simulink model "Simulator_hquad_LQR_trajectory"  (Simulink 7.6)
settings: Solver=ode3  StartTime=0.0  StopTime=40  FixedStep=Ts  RelTol=1e-3
values from neighbouring files (symbols this model uses):
  g = 9.8065    [kostas_malakies.mat]    (also in kostas_malakies2.mat; load_PMModel.m = 9.81; main_last.m; matlab.mat)
  mass = 0.66    [kostas_malakies.mat]    (also in kostas_malakies2.mat; load_PMModel.m = 0.687; main_last.m)
  Ts = 0.02    [kostas_malakies.mat]    (also in kostas_malakies2.mat; main.m; main_last.m; matlab.mat = 0.08)
  Ts_slow = 0.02    [kostas_malakies.mat]    (also in kostas_malakies2.mat; main.m; main_last.m)
  yaw0 = 0    [kostas_malakies.mat]    (also in kostas_malakies2.mat; main.m; main_last.m; matlab.mat = -0.0873)
libraries: simulink x14, Hqaud_model_LIB_SI x5, Hquad_control_LIB_LQR x5, sdolib x4
settings Model: Creator=andi  LastModifiedBy=burrimi
settings DebuggingCC: InheritedTsInSrcMsg=none  StrictBusMsg=Warning
settings SFSimCC: SimParseCustomCode=off

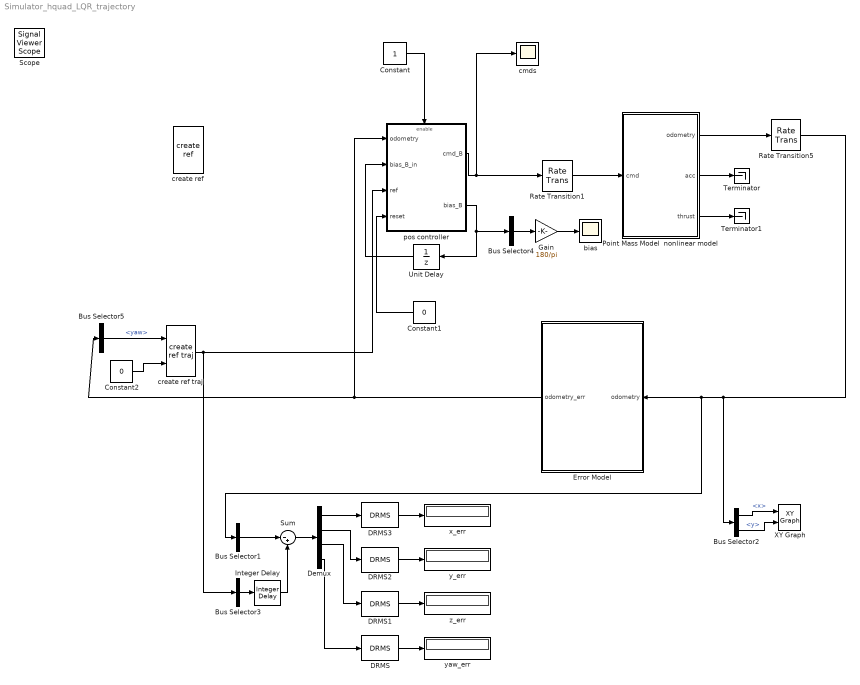
== system Simulator_hquad_LQR_trajectory ==
  Bus Selector1 : BusSelector  OutputSignals=pos.x,pos.y,pos.z,rpy.yaw  OutputAsBus=on
  Bus Selector2 : BusSelector  OutputSignals=pos.x,pos.y
  Bus Selector3 : BusSelector  OutputSignals=x_ref,y_ref,z_ref,yaw_ref  OutputAsBus=on
  Bus Selector4 : BusSelector  OutputSignals=pitch_bias,roll_bias,thrust_bias  OutputAsBus=on
  Bus Selector5 : BusSelector  OutputSignals=rpy.yaw
  Constant : Constant
  Constant1 : Constant  Value=0
  Constant2 : Constant  Value=0
  DRMS{,1..3} (4 alike) : sdolib/RMS Blocks/DRMS  SystemSampleTime=-1  Ts=Ts
  Demux : Demux
  Error Model : Subsystem
  Gain : Gain  Gain=180/pi
  Integer Delay : simulink/Discrete/Integer Delay  NumDelays=3  vinit=0.0  samptime=-1
  Point Mass Model  nonlinear model : Subsystem  AncestorBlock="Hqaud_model_LIB_SI/Point Mass Model  nonlinear model"
  Rate Transition1 : RateTransition
  Rate Transition5 : RateTransition  OutPortSampleTime=Ts
  Sum : Sum  Inputs=|-+
  Terminator : Terminator
  Terminator1 : Terminator
  Unit Delay : UnitDelay  SampleTime=-1
  XY Graph : simulink/Sinks/XY Graph  SystemSampleTime=-1  xmin=-2  xmax=2  ymin=-2  ymax=2  st=-1
  bias : Scope
      settings: TimeRange=39.996  YMin=-0.07  YMax=0.05  SaveName=ScopeData14
  cmds : Scope
      settings: TimeRange=40  YMin=-0.5  YMax=0.5
  create ref : Hquad_control_LIB_LQR/create ref  SystemSampleTime=-1
  create ref traj : Hquad_control_LIB_LQR/create ref traj  SystemSampleTime=-1
  pos controller : Subsystem  AncestorBlock=Hquad_control_LIB_LQR/pos controller
  x_err : Display
  y_err : Display
  yaw_err : Display
  z_err : Display
  Scope : SignalViewerScope  IOType=viewer  LegendLocations="321.25       180.625         123.5       128.125"  RefreshTime=0.035000
      settings: ShowLegends=on
  wires:
  Point Mass Model  nonlinear model/3("thrust   ") -> Terminator1/1
  pos controller/1(cmd_B) -> cmds/1, Rate Transition1/1
  Constant/1 -> pos controller/Enable
  Point Mass Model  nonlinear model/2(acc) -> Terminator/1
  Constant1/1 -> pos controller/4(reset)
  Point Mass Model  nonlinear model/1(odometry) -> Rate Transition5/1
  Error Model/1(odometry_err) -> Bus Selector5/1, pos controller/1(odometry)
  Rate Transition5/1 -> Bus Selector2/1, Error Model/1(odometry), Bus Selector1/1
  Bus Selector1/1 -> Sum/1
  Sum/1 -> Demux/1
  Demux/1 -> DRMS3/1
  Demux/2 -> DRMS2/1
  Demux/3 -> DRMS1/1
  Demux/4 -> DRMS/1
  DRMS/1 -> yaw_err/1
  DRMS1/1 -> z_err/1
  DRMS2/1 -> y_err/1
  DRMS3/1 -> x_err/1
  Rate Transition1/1 -> Point Mass Model  nonlinear model/1(cmd)
  Bus Selector3/1 -> Integer Delay/1
  Bus Selector5/1 -> create ref traj/1  "<yaw>"
  pos controller/2(bias_B) -> Unit Delay/1, Bus Selector4/1
  Bus Selector4/1 -> Gain/1
  Gain/1 -> bias/1
  Unit Delay/1 -> pos controller/2(bias_B_in)
  create ref traj/1 -> Bus Selector3/1, pos controller/3(ref)
  Bus Selector2/1 -> XY Graph/1  "<x>"
  Bus Selector2/2 -> XY Graph/2  "<y>"
  Integer Delay/1 -> Sum/2
  Constant2/1 -> create ref traj/2

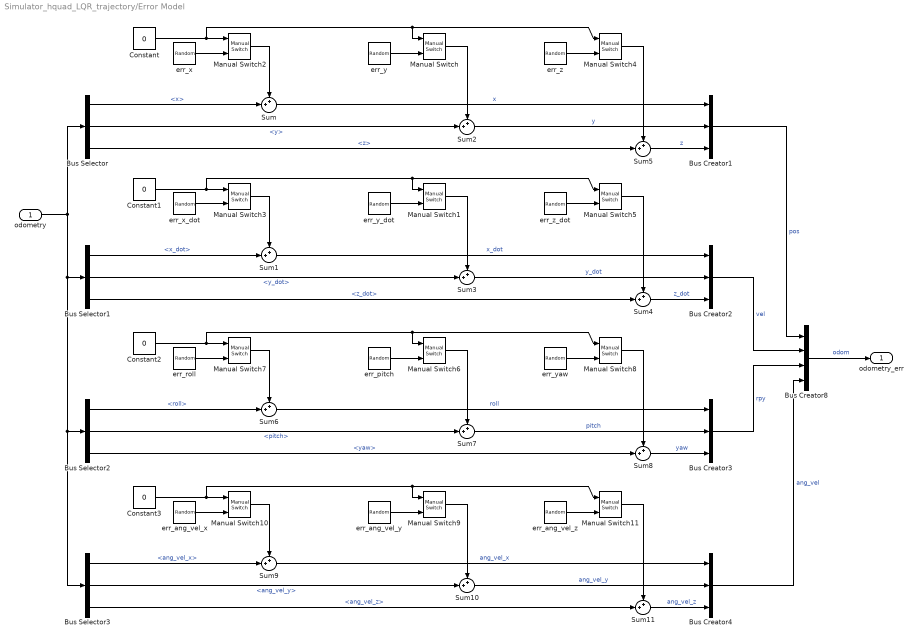
== system Simulator_hquad_LQR_trajectory/Error Model ==
  odometry : Inport
  Bus Creator{1..4} (4 alike) : BusCreator  Inputs=3
  Bus Creator8 : BusCreator
  Bus Selector : BusSelector  OutputSignals=pos.x,pos.y,pos.z
  Bus Selector1 : BusSelector  OutputSignals=vel.x_dot,vel.y_dot,vel.z_dot
  Bus Selector2 : BusSelector  OutputSignals=rpy.roll,rpy.pitch,rpy.yaw
  Bus Selector3 : BusSelector  OutputSignals=ang_vel.ang_vel_x,ang_vel.ang_vel_y,ang_vel.ang_vel_z
  Constant{,1..3} (4 alike) : Constant  Value=0
  Manual Switch{,1..11} (12 alike) : simulink/Signal Routing/Manual Switch  SystemSampleTime=-1  sw=1  action=0  varsize=off
  Sum{,1..11} (12 alike) : Sum  Inputs=++|  SampleTime=Ts_slow
  err_ang_vel_x : RandomNumber  Variance=0.0001  SampleTime=Ts_slow
  err_ang_vel_y : RandomNumber  Variance=0.0001  SampleTime=Ts_slow
  err_ang_vel_z : RandomNumber  Variance=0.0001  SampleTime=Ts_slow
  err_pitch : RandomNumber  Variance=0.0001  SampleTime=Ts_slow
  err_roll : RandomNumber  Variance=0.0001  SampleTime=Ts_slow
  err_x : RandomNumber  Variance=0.000707  SampleTime=Ts_slow
  err_x_dot : RandomNumber  Variance=0.0001  SampleTime=Ts_slow
  err_y : RandomNumber  Variance=0.000707  SampleTime=Ts_slow
  err_y_dot : RandomNumber  Variance=0.0001  SampleTime=Ts_slow
  err_yaw : RandomNumber  Variance=0.0001  SampleTime=Ts_slow
  err_z : RandomNumber  Variance=0.000707  SampleTime=Ts_slow
  err_z_dot : RandomNumber  Variance=0.0001  SampleTime=Ts_slow
  odometry_err : Outport
  wires:
  err_z/1 -> Manual Switch4/2
  Manual Switch4/1 -> Sum5/1
  err_y/1 -> Manual Switch/2
  Manual Switch/1 -> Sum2/1
  err_x/1 -> Manual Switch2/2
  Manual Switch2/1 -> Sum/1
  Sum/1 -> Bus Creator1/1  "x"
  Bus Creator1/1 -> Bus Creator8/1  "pos"
  Sum2/1 -> Bus Creator1/2  "y"
  Sum5/1 -> Bus Creator1/3  "z"
  odometry/1 -> Bus Selector/1, Bus Selector2/1, Bus Selector3/1, Bus Selector1/1
  Bus Selector/1 -> Sum/2  "<x>"
  Bus Selector/2 -> Sum2/2  "<y>"
  Bus Selector/3 -> Sum5/2  "<z>"
  Constant/1 -> Manual Switch2/1, Manual Switch/1, Manual Switch4/1
  err_z_dot/1 -> Manual Switch5/2
  Manual Switch5/1 -> Sum4/1
  err_y_dot/1 -> Manual Switch1/2
  Manual Switch1/1 -> Sum3/1
  err_x_dot/1 -> Manual Switch3/2
  Manual Switch3/1 -> Sum1/1
  Sum1/1 -> Bus Creator2/1  "x_dot"
  Sum3/1 -> Bus Creator2/2  "y_dot"
  Sum4/1 -> Bus Creator2/3  "z_dot"
  Bus Selector1/1 -> Sum1/2  "<x_dot>"
  Bus Selector1/2 -> Sum3/2  "<y_dot>"
  Bus Selector1/3 -> Sum4/2  "<z_dot>"
  Constant1/1 -> Manual Switch3/1, Manual Switch1/1, Manual Switch5/1
  Bus Creator2/1 -> Bus Creator8/2  "vel"
  err_yaw/1 -> Manual Switch8/2
  Manual Switch8/1 -> Sum8/1
  err_pitch/1 -> Manual Switch6/2
  Manual Switch6/1 -> Sum7/1
  err_roll/1 -> Manual Switch7/2
  Manual Switch7/1 -> Sum6/1
  Sum6/1 -> Bus Creator3/1  "roll"
  Sum7/1 -> Bus Creator3/2  "pitch"
  Sum8/1 -> Bus Creator3/3  "yaw"
  Bus Selector2/1 -> Sum6/2  "<roll>"
  Bus Selector2/2 -> Sum7/2  "<pitch>"
  Bus Selector2/3 -> Sum8/2  "<yaw>"
  Constant2/1 -> Manual Switch7/1, Manual Switch6/1, Manual Switch8/1
  Bus Creator3/1 -> Bus Creator8/3  "rpy"
  err_ang_vel_z/1 -> Manual Switch11/2
  Manual Switch11/1 -> Sum11/1
  err_ang_vel_y/1 -> Manual Switch9/2
  Manual Switch9/1 -> Sum10/1
  err_ang_vel_x/1 -> Manual Switch10/2
  Manual Switch10/1 -> Sum9/1
  Sum9/1 -> Bus Creator4/1  "ang_vel_x"
  Sum10/1 -> Bus Creator4/2  "ang_vel_y"
  Sum11/1 -> Bus Creator4/3  "ang_vel_z"
  Bus Selector3/1 -> Sum9/2  "<ang_vel_x>"
  Bus Selector3/2 -> Sum10/2  "<ang_vel_y>"
  Bus Selector3/3 -> Sum11/2  "<ang_vel_z>"
  Constant3/1 -> Manual Switch10/1, Manual Switch9/1, Manual Switch11/1
  Bus Creator4/1 -> Bus Creator8/4  "ang_vel"
  Bus Creator8/1 -> odometry_err/1  "odom"

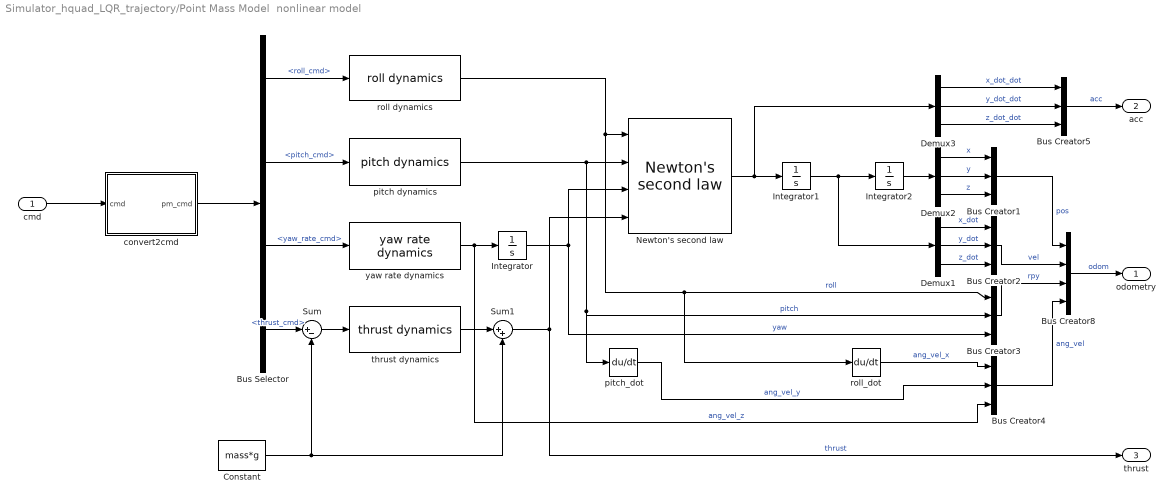
== system Simulator_hquad_LQR_trajectory/Point Mass Model  nonlinear model ==
  cmd : Inport
  Bus Creator{1..5} (5 alike) : BusCreator  Inputs=3
  Bus Creator8 : BusCreator
  Bus Selector : BusSelector  OutputSignals=roll_cmd,pitch_cmd,yaw_rate_cmd,thrust_cmd
  Constant : Constant  Value=mass*g
  Demux1 : Demux  Outputs=3
  Demux2 : Demux  Outputs=3
  Demux3 : Demux  Outputs=3
  Integrator : Integrator  InitialCondition=yaw0
  Integrator1 : Integrator
  Integrator2 : Integrator
  "Newton's second law  " : Hqaud_model_LIB_SI/Newton's second law    SystemSampleTime=-1
  Sum : Sum  Inputs=|+-
  Sum1 : Sum  Inputs=|++
  convert2cmd : Subsystem
  "pitch dynamics  " : Hqaud_model_LIB_SI/pitch dynamics    SystemSampleTime=-1
  pitch_dot : Derivative
  roll dynamics : Hqaud_model_LIB_SI/roll dynamics  SystemSampleTime=-1
  roll_dot : Derivative
  "thrust dynamics  " : Hqaud_model_LIB_SI/thrust dynamics    SystemSampleTime=-1
  "yaw rate dynamics  " : Hqaud_model_LIB_SI/yaw rate dynamics    SystemSampleTime=-1
  odometry : Outport
  acc : Outport  Port=2
  "thrust   " : Outport  Port=3  PortDimensions=1
  wires:
  convert2cmd/1(pm_cmd) -> Bus Selector/1
  Bus Selector/1 -> roll dynamics/1  "<roll_cmd>"
  "yaw rate dynamics  "/1 -> Integrator/1, Bus Creator4/3  "ang_vel_z"
  Integrator/1 -> "Newton's second law  "/3, Bus Creator3/3  "yaw"
  "thrust dynamics  "/1 -> Sum1/1
  "pitch dynamics  "/1 -> "Newton's second law  "/2, Bus Creator3/2, pitch_dot/1  "pitch"
  roll dynamics/1 -> "Newton's second law  "/1, Bus Creator3/1, roll_dot/1  "roll"
  "Newton's second law  "/1 -> Integrator1/1, Demux3/1
  Integrator1/1 -> Integrator2/1, Demux1/1
  Integrator2/1 -> Demux2/1
  Demux2/2 -> Bus Creator1/2  "y"
  Constant/1 -> Sum/2, Sum1/2
  Sum/1 -> "thrust dynamics  "/1
  Bus Selector/4 -> Sum/1  "<thrust_cmd>"
  cmd/1 -> convert2cmd/1(cmd)
  Bus Selector/2 -> "pitch dynamics  "/1  "<pitch_cmd>"
  Bus Selector/3 -> "yaw rate dynamics  "/1  "<yaw_rate_cmd>"
  Bus Creator4/1 -> Bus Creator8/4  "ang_vel"
  Bus Creator3/1 -> Bus Creator8/3  "rpy"
  Bus Creator2/1 -> Bus Creator8/2  "vel"
  Bus Creator1/1 -> Bus Creator8/1  "pos"
  Bus Creator8/1 -> odometry/1  "odom"
  Demux2/3 -> Bus Creator1/3  "z"
  Demux2/1 -> Bus Creator1/1  "x"
  Demux1/1 -> Bus Creator2/1  "x_dot"
  Demux1/2 -> Bus Creator2/2  "y_dot"
  Demux1/3 -> Bus Creator2/3  "z_dot"
  Bus Creator5/1 -> acc/1  "acc"
  Demux3/1 -> Bus Creator5/1  "x_dot_dot"
  Demux3/2 -> Bus Creator5/2  "y_dot_dot"
  Demux3/3 -> Bus Creator5/3  "z_dot_dot"
  Sum1/1 -> "Newton's second law  "/4, "thrust   "/1  "thrust"
  roll_dot/1 -> Bus Creator4/1  "ang_vel_x"
  pitch_dot/1 -> Bus Creator4/2  "ang_vel_y"

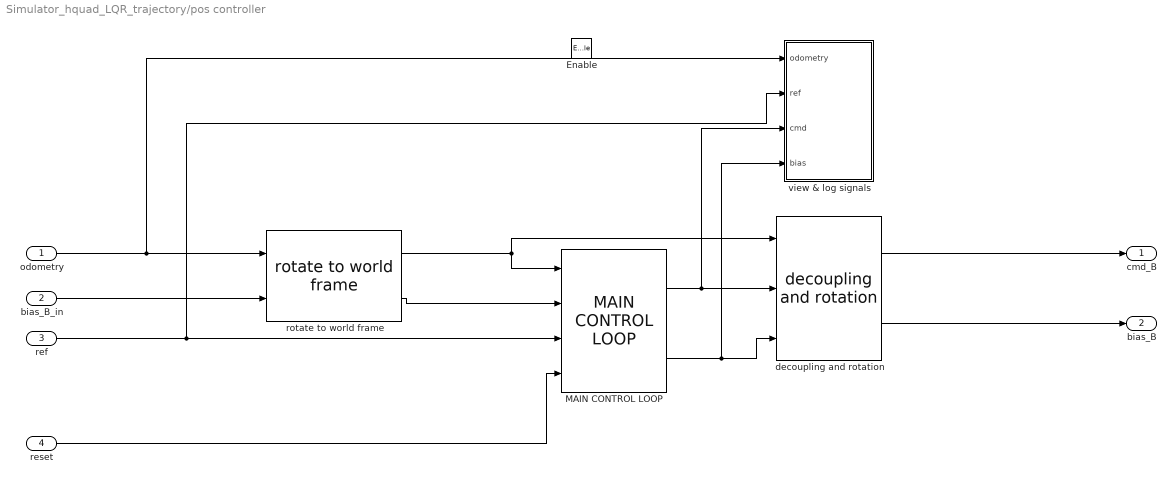
== system Simulator_hquad_LQR_trajectory/pos controller ==
  odometry : Inport
  bias_B_in : Inport  Port=2
  ref : Inport  Port=3
  reset : Inport  Port=4
  Enable : EnablePort  StatesWhenEnabling=reset
  MAIN CONTROL LOOP : Hquad_control_LIB_LQR/MAIN CONTROL LOOP  Priority=2  SystemSampleTime=-1
  decoupling and rotation : Hquad_control_LIB_LQR/decoupling and rotation  Priority=3  SystemSampleTime=-1
  rotate to world frame : Hquad_control_LIB_LQR/rotate to world frame  Priority=1  SystemSampleTime=-1
  view & log signals : Subsystem  AncestorBlock=Hquad_control_LIB_LQR/view & log signals
  cmd_B : Outport
  bias_B : Outport  Port=2
  wires:
  bias_B_in/1 -> rotate to world frame/2
  rotate to world frame/2 -> MAIN CONTROL LOOP/2
  decoupling and rotation/2 -> bias_B/1
  decoupling and rotation/1 -> cmd_B/1
  MAIN CONTROL LOOP/2 -> decoupling and rotation/3, view & log signals/4(bias)
  rotate to world frame/1 -> MAIN CONTROL LOOP/1, decoupling and rotation/1
  ref/1 -> MAIN CONTROL LOOP/3, view & log signals/2(ref)
  reset/1 -> MAIN CONTROL LOOP/4
  odometry/1 -> rotate to world frame/1, view & log signals/1(odometry)
  MAIN CONTROL LOOP/1 -> decoupling and rotation/2, view & log signals/3(cmd)

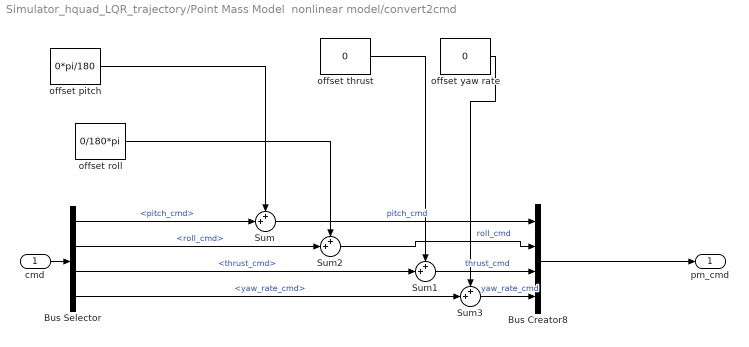
== system Simulator_hquad_LQR_trajectory/Point Mass Model  nonlinear model/convert2cmd ==
  cmd : Inport
  Bus Creator8 : BusCreator
  Bus Selector : BusSelector  OutputSignals=pitch_cmd,roll_cmd,thrust_cmd,yaw_rate_cmd
  Sum{,1..3} (4 alike) : Sum  Inputs=++|
  offset pitch : Constant  Value=0*pi/180
  offset roll : Constant  Value=0/180*pi
  offset thrust : Constant  Value=0
  offset yaw rate : Constant  Value=0
  pm_cmd : Outport
  wires:
  cmd/1 -> Bus Selector/1
  Bus Creator8/1 -> pm_cmd/1
  offset pitch/1 -> Sum/1
  Bus Selector/1 -> Sum/2  "<pitch_cmd>"
  Sum/1 -> Bus Creator8/1  "pitch_cmd"
  Bus Selector/3 -> Sum1/2  "<thrust_cmd>"
  Sum1/1 -> Bus Creator8/3  "thrust_cmd"
  offset thrust/1 -> Sum1/1
  Sum2/1 -> Bus Creator8/2  "roll_cmd"
  Bus Selector/2 -> Sum2/2  "<roll_cmd>"
  offset roll/1 -> Sum2/1
  Sum3/1 -> Bus Creator8/4  "yaw_rate_cmd"
  Bus Selector/4 -> Sum3/2  "<yaw_rate_cmd>"
  offset yaw rate/1 -> Sum3/1

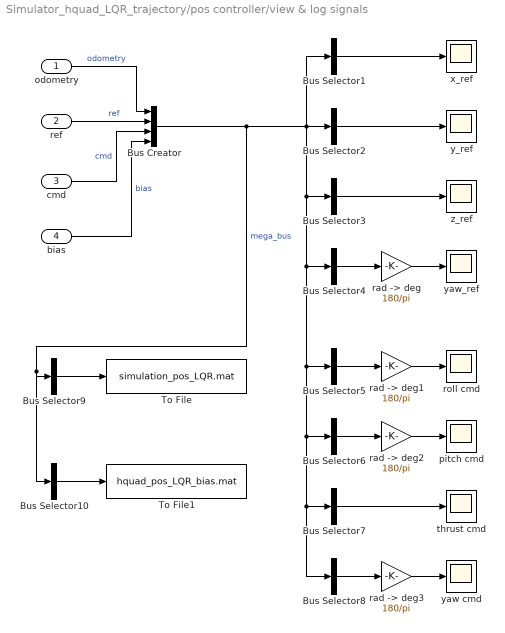
== system Simulator_hquad_LQR_trajectory/pos controller/view & log signals ==
  odometry : Inport
  ref : Inport  Port=2
  cmd : Inport  Port=3
  bias : Inport  Port=4
  Bus Creator : BusCreator
  Bus Selector1 : BusSelector  OutputSignals=odometry.pos.x,odometry.vel.x_dot,ref.x_ref,ref.x_dot_ref  OutputAsBus=on
  Bus Selector10 : BusSelector  OutputSignals=bias.pitch_bias,bias.roll_bias,bias.thrust_bias,bias.yaw_rate_bias  OutputAsBus=on
  Bus Selector2 : BusSelector  OutputSignals=odometry.pos.y,odometry.vel.y_dot,ref.y_ref,ref.y_dot_ref  OutputAsBus=on
  Bus Selector3 : BusSelector  OutputSignals=odometry.pos.z,odometry.vel.z_dot,ref.z_ref,ref.z_dot_ref  OutputAsBus=on
  Bus Selector4 : BusSelector  OutputSignals=odometry.rpy.yaw,odometry.ang_vel.ang_vel_z,ref.yaw_ref,ref.yaw_dot_ref  OutputAsBus=on
  Bus Selector5 : BusSelector  OutputSignals=odometry.rpy.roll,odometry.ang_vel.ang_vel_x,cmd.roll_cmd  OutputAsBus=on
  Bus Selector6 : BusSelector  OutputSignals=odometry.rpy.pitch,odometry.ang_vel.ang_vel_y,cmd.pitch_cmd  OutputAsBus=on
  Bus Selector7 : BusSelector  OutputSignals=odometry.pos.z,ref.z_ref,cmd.thrust_cmd  OutputAsBus=on
  Bus Selector8 : BusSelector  OutputSignals=odometry.rpy.yaw,odometry.ang_vel.ang_vel_z,cmd.yaw_rate_cmd  OutputAsBus=on
  Bus Selector9 : BusSelector  OutputSignals=odometry.pos.x,odometry.vel.x_dot,odometry.rpy.pitch,ref.x_ref,cmd.pitch_cmd,odometry.pos.y,odometry.vel.y_dot,odometry.rpy.roll,ref.y_ref,cmd.roll_cmd,odometry.pos.z,odometry.vel.z_dot,ref.z_ref,cmd.thrust_cmd,odometry.rpy.yaw,odometry.ang_vel.ang_vel_z,ref.yaw_ref,cmd.yaw_rate_cmd  OutputAsBus=on
  To File : ToFile  Filename=simulation_pos_LQR.mat  MatrixName=simulation_pos_LQR
  To File1 : ToFile  Filename=hquad_pos_LQR_bias.mat  MatrixName=hquad_pos_LQR_bias
  pitch cmd : Scope
      settings: YMin=-15  YMax=15  SaveName=ScopeData2
  rad -> deg{,1..3} (4 alike) : Gain  Gain=180/pi
  roll cmd : Scope
      settings: YMin=-100  YMax=100
  thrust cmd : Scope
      settings: YMin=-3  YMax=3  SaveName=ScopeData11
  x_ref : Scope
      settings: TimeRange=40  YMin=-1.5  YMax=1.5  SaveName=ScopeData3
  y_ref : Scope
      settings: TimeRange=40  YMin=-0.75  YMax=2.75
  yaw cmd : Scope
      settings: YMin=-60  YMax=-0  SaveName=ScopeData10
  yaw_ref : Scope
      settings: TimeRange=39.996  YMin=-1.5  YMax=8.5  SaveName=ScopeData8
  z_ref : Scope
      settings: TimeRange=40  YMin=-21  YMax=1  SaveName=ScopeData5
  wires:
  Bus Selector10/1 -> To File1/1
  bias/1 -> Bus Creator/4  "bias"
  Bus Selector8/1 -> "rad -> deg3"/1
  Bus Selector6/1 -> "rad -> deg2"/1
  Bus Selector5/1 -> "rad -> deg1"/1
  Bus Selector7/1 -> thrust cmd/1
  Bus Selector4/1 -> "rad -> deg"/1
  Bus Selector3/1 -> z_ref/1
  Bus Selector2/1 -> y_ref/1
  Bus Selector1/1 -> x_ref/1
  Bus Creator/1 -> Bus Selector10/1, Bus Selector9/1, Bus Selector8/1, Bus Selector7/1, Bus Selector6/1, Bus Selector5/1, Bus Selector4/1, Bus Selector3/1, Bus Selector2/1, Bus Selector1/1  "mega_bus"
  cmd/1 -> Bus Creator/3  "cmd"
  ref/1 -> Bus Creator/2  "ref"
  odometry/1 -> Bus Creator/1  "odometry"
  "rad -> deg3"/1 -> yaw cmd/1
  "rad -> deg2"/1 -> pitch cmd/1
  "rad -> deg1"/1 -> roll cmd/1
  "rad -> deg"/1 -> yaw_ref/1
  Bus Selector9/1 -> To File/1
